simulink model "project2_ex1"  (R2017a)
settings: Solver=VariableStepAuto  StartTime=0.0  StopTime=10.0  RelTol=1e-3
libraries: simulink x1
settings Model: Creator=ignacio  LastModifiedBy=ignacio

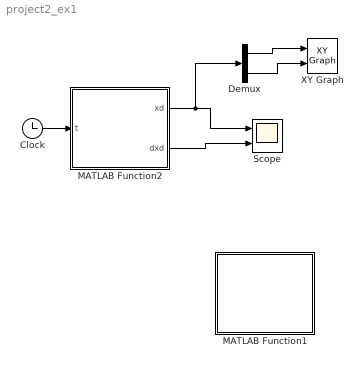
== system project2_ex1 ==
  Clock : Clock
  Demux : Demux  Outputs=3
  MATLAB Function1 : MATLAB Function  TreatAsAtomicUnit=on
  MATLAB Function2 : MATLAB Function  TreatAsAtomicUnit=on
  Scope : Scope  NumInputPorts=2
  XY Graph : simulink/Sinks/XY Graph  xmin=-1  xmax=1  ymin=-1  ymax=1  st=-1
  wires:
  Clock/1 -> MATLAB Function2/1(t)
  MATLAB Function2/1(xd) -> Demux/1, Scope/1
  MATLAB Function2/2(dxd) -> Scope/2
  Demux/1 -> XY Graph/1
  Demux/3 -> XY Graph/2

== matlab function project2_ex1/MATLAB Function1 ==
function kine
xd = xd1(t);
dxd = dx_xd1(t);

== matlab function project2_ex1/MATLAB Function2 ==
  data: t input; xd output; dxd output
function [xd, dxd] = trajectories(t)
xd = xd1(t);
dxd = dx_xd1(t);
